simulink model "Lab1B_Task1"  (R2019b)
settings: Solver=FixedStepAuto  StartTime=0.0  StopTime=50.0  FixedStep=1e-1  RelTol=1e-3
settings Model: Creator=sinow  LastModifiedBy=sinow

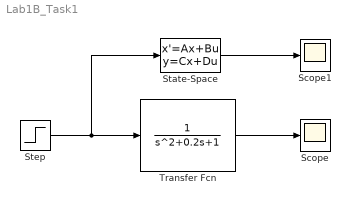
== system Lab1B_Task1 ==
  Scope : Scope
  Scope1 : Scope
  State-Space : StateSpace  A=[0 1; -1 -0.2]  B=[0; 1]  C=[1 0]  D=0  InitialCondition=0
  Step : Step  Time=0  SampleTime=0
  Transfer Fcn : TransferFcn  Denominator=[1 0.2 1]
  wires:
  Step/1 -> State-Space/1, Transfer Fcn/1
  Transfer Fcn/1 -> Scope/1
  State-Space/1 -> Scope1/1
